simulink model "QPTest5"  (R2021a)
settings: Solver=ode45  StartTime=0.0  StopTime=20  FixedStep=Control_timestep  RelTol=1e-3  AbsTol=1e-6
undefined symbols (not defined in the file): Matlab_version, NXMotion, NXMotion_controltimestep, NXMotion_model, NXMotion_model_n, NXMotion_n, NXMotion_solution, NXMotion_solution_n, Plant_inputs_num, Plant_outputs_num
libraries: simulink x1
(part 1 of 3)
settings Model: ExtModeTrigMode=oneshot  ExtModeArmWhenConnect=off  Creator=djyun  LastModifiedBy=Bec
settings SolverCC: AutoScaleAbsTol=off  AlgebraicLoopSolver=TrustRegion
settings DataIOCC: SaveFormat=Array  SignalLoggingSaveFormat=ModelDataLogs  ReturnWorkspaceOutputs=off
settings OptimizationCC: BooleanDataType=off  InitFltsAndDblsToZero=on  LifeSpan=inf
settings DebuggingCC: SaveWithParameterizedLinksMsg=none  UnderspecifiedInitializationDetection=Classic  MergeDetectMultiDrivingBlocksExec=none  SignalResolutionControl=TryResolveAllWithWarning  MultiTaskDSMMsg=warning  MultiTaskCondExecSysMsg=none  FcnCallInpInsideContextMsg=warning  SFUnexpectedBacktrackingDiag=warning  SFNoUnconditionalDefaultTransitionDiag=warning  SFExecutionAtInitializationDiag=none  SFMachineParentedDataDiag=warning  ArithmeticOperatorsInVariantConditions=warning
settings HardwareCC: ProdBitPerPointer=32  ProdBitPerSizeT=32  ProdBitPerPtrDiffT=32  ProdLargestAtomicFloat=None  ProdIntDivRoundTo=Undefined  ProdEndianess=Unspecified  ProdWordSize=32  ProdHWDeviceType=32-bit Generic  TargetUnknown=on
settings ModelReferenceCC: PropagateSignalLabelsOutOfModel=off
settings RTWCC: TemplateMakefile=grt_unix.tmf
settings CodeAppCC: StateflowObjectComments=on
settings GRTTargetCC: TargetFcnLib=ansi_tfl_tmw.mat  TargetLangStandard=C89/C90 (ANSI)  ModelReferenceCompliant=off  CombineOutputUpdateFcns=off  MatFileLogging=off  GRTInterface=on
settings ConfigComp: CovMetricSettings=dw  CovSaveCumulativeToWorkspaceVar=on  CovSaveSingleToWorkspaceVar=on

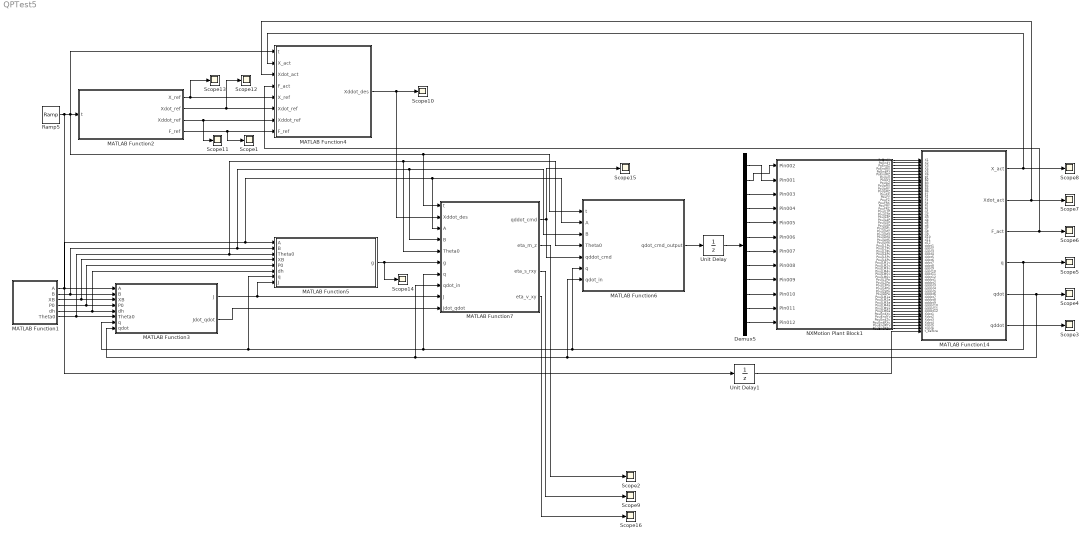
== system QPTest5 ==
  Demux5 : Demux  Outputs=12
  MATLAB Function1 : MATLAB Function  TreatAsAtomicUnit=on
  MATLAB Function14 : MATLAB Function  TreatAsAtomicUnit=on
  MATLAB Function2 : MATLAB Function  TreatAsAtomicUnit=on
  MATLAB Function3 : MATLAB Function  TreatAsAtomicUnit=on
  MATLAB Function4 : MATLAB Function  TreatAsAtomicUnit=on
  MATLAB Function5 : MATLAB Function  TreatAsAtomicUnit=on
  MATLAB Function6 : MATLAB Function  TreatAsAtomicUnit=on
  MATLAB Function7 : MATLAB Function  TreatAsAtomicUnit=on
  NXMotion Plant Block1 : Subsystem
      mask Display: image(imread('NXMOTION_Logo_Client.TIF'))
  Ramp5 : simulink/Sources/Ramp  slope=1  start=0  InitialOutput=0
  Scope{1..16} (16 alike) : Scope
  Unit Delay : UnitDelay  InitialCondition=zeros(12,1)  SampleTime=1e-3  HasFrameUpgradeWarning=on
  Unit Delay1 : UnitDelay  InitialCondition=zeros(1,1)  SampleTime=1e-3  HasFrameUpgradeWarning=on
  wires:
  MATLAB Function2/1(X_ref) -> MATLAB Function4/5(X_ref), Scope13/1
  MATLAB Function2/2(Xdot_ref) -> MATLAB Function4/6(Xdot_ref), Scope12/1
  MATLAB Function2/3(Xddot_ref) -> MATLAB Function4/7(Xddot_ref), Scope11/1
  MATLAB Function7/1(qddot_cmd) -> Scope15/1, MATLAB Function6/5(qddot_cmd)
  MATLAB Function2/4(F_ref) -> MATLAB Function4/8(F_ref), Scope1/1
  MATLAB Function3/1(J) -> MATLAB Function5/8(J), MATLAB Function7/9(J)
  MATLAB Function3/2(Jdot_qdot) -> MATLAB Function7/10(Jdot_qdot)
  MATLAB Function4/1(Xddot_des) -> Scope10/1, MATLAB Function7/2(Xddot_des)
  MATLAB Function5/1(g) -> Scope14/1, MATLAB Function7/6(g)
  MATLAB Function1/1(A) -> MATLAB Function3/1(A), MATLAB Function6/2(A), MATLAB Function7/3(A), MATLAB Function5/1(A)
  MATLAB Function1/2(B) -> MATLAB Function6/3(B), MATLAB Function7/4(B), MATLAB Function5/2(B), MATLAB Function3/2(B)
  MATLAB Function1/3(XB) -> MATLAB Function5/4(XB), MATLAB Function3/3(XB)
  MATLAB Function1/4(P0) -> MATLAB Function5/5(P0), MATLAB Function3/4(P0)
  MATLAB Function1/5(dh) -> MATLAB Function5/6(dh), MATLAB Function3/5(dh)
  MATLAB Function1/6(Theta0) -> MATLAB Function6/4(Theta0), MATLAB Function7/5(Theta0), MATLAB Function5/3(Theta0), MATLAB Function3/6(Theta0)
  MATLAB Function6/1(qdot_cmd_output) -> Unit Delay/1
  Unit Delay/1 -> Demux5/1
  MATLAB Function14/1(X_act) -> Scope8/1, MATLAB Function4/2(X_act)
  MATLAB Function14/2(Xdot_act) -> Scope7/1, MATLAB Function4/3(Xdot_act)
  MATLAB Function14/3(F_act) -> Scope6/1, MATLAB Function4/4(F_act)
  MATLAB Function14/4(q) -> MATLAB Function3/7(q), MATLAB Function5/7(q), MATLAB Function7/7(q), MATLAB Function6/6(q), Scope5/1
  MATLAB Function14/5(qdot) -> MATLAB Function7/8(qdot_in), MATLAB Function3/8(qdot), MATLAB Function6/7(qdot_in), Scope4/1
  MATLAB Function14/6(qddot) -> Scope3/1
  Demux5/3 -> NXMotion Plant Block1/3(Pin003)
  Demux5/4 -> NXMotion Plant Block1/4(Pin004)
  Demux5/5 -> NXMotion Plant Block1/5(Pin005)
  Demux5/6 -> NXMotion Plant Block1/6(Pin006)
  Demux5/7 -> NXMotion Plant Block1/7(Pin007)
  Demux5/8 -> NXMotion Plant Block1/8(Pin008)
  Demux5/9 -> NXMotion Plant Block1/9(Pin009)
  Demux5/10 -> NXMotion Plant Block1/10(Pin010)
  Demux5/11 -> NXMotion Plant Block1/11(Pin011)
  Demux5/12 -> NXMotion Plant Block1/12(Pin012)
  Demux5/2 -> NXMotion Plant Block1/1(Pin002)
  Demux5/1 -> NXMotion Plant Block1/2(Pin001)
  Ramp5/1 -> Unit Delay1/1, MATLAB Function6/1(t), MATLAB Function7/1(t), MATLAB Function2/1(t), MATLAB Function4/1(t)
  NXMotion Plant Block1/1("PoEndX   ") -> MATLAB Function14/1(X1)
  NXMotion Plant Block1/2("PoEndY   ") -> MATLAB Function14/2(X2)
  NXMotion Plant Block1/3("PoEndZ   ") -> MATLAB Function14/3(X3)
  NXMotion Plant Block1/4("PoEndRX  ") -> MATLAB Function14/4(X4)
  NXMotion Plant Block1/5("PoEndRY  ") -> MATLAB Function14/5(X5)
  NXMotion Plant Block1/6("PoEndRZ  ") -> MATLAB Function14/6(X6)
  NXMotion Plant Block1/7("PoUpX    ") -> MATLAB Function14/7(B1)
  NXMotion Plant Block1/8("PoUpY    ") -> MATLAB Function14/8(B2)
  NXMotion Plant Block1/9("PoUpZ    ") -> MATLAB Function14/9(B3)
  NXMotion Plant Block1/10("PoUpRX   ") -> MATLAB Function14/10(B4)
  NXMotion Plant Block1/11("PoUpRY   ") -> MATLAB Function14/11(B5)
  NXMotion Plant Block1/12("PoUpRZ   ") -> MATLAB Function14/12(B6)
  NXMotion Plant Block1/13("PouFX    ") -> MATLAB Function14/13(F1)
  NXMotion Plant Block1/14("PouFY    ") -> MATLAB Function14/14(F2)
  NXMotion Plant Block1/15("PouFZ    ") -> MATLAB Function14/15(F3)
  NXMotion Plant Block1/16("PouFRX   ") -> MATLAB Function14/16(F4)
  NXMotion Plant Block1/17("PouFRY   ") -> MATLAB Function14/17(F5)
  NXMotion Plant Block1/18("PouFRZ   ") -> MATLAB Function14/18(F6)
  NXMotion Plant Block1/19("PouJL1P  ") -> MATLAB Function14/19(q1)
  NXMotion Plant Block1/20("PouJL2P  ") -> MATLAB Function14/20(q2)
  NXMotion Plant Block1/21("PouJL3P  ") -> MATLAB Function14/21(q3)
  NXMotion Plant Block1/22("PouJL4P  ") -> MATLAB Function14/22(q4)
  NXMotion Plant Block1/23("PouJL5P  ") -> MATLAB Function14/23(q5)
  NXMotion Plant Block1/24("PouJL6P  ") -> MATLAB Function14/24(q6)
  NXMotion Plant Block1/25("PouJLM1  ") -> MATLAB Function14/25(q7)
  NXMotion Plant Block1/26("PouJLM2  ") -> MATLAB Function14/26(q8)
  NXMotion Plant Block1/27("PouJLM3  ") -> MATLAB Function14/27(q9)
  NXMotion Plant Block1/28("PouJLM4  ") -> MATLAB Function14/28(q10)
  NXMotion Plant Block1/29("PouJLM5  ") -> MATLAB Function14/29(q11)
  NXMotion Plant Block1/30("PouJLM6  ") -> MATLAB Function14/30(q12)
  NXMotion Plant Block1/31("PouJL1Pv ") -> MATLAB Function14/31(qdot1)
  NXMotion Plant Block1/32("PouJL2Pv ") -> MATLAB Function14/32(qdot2)
  NXMotion Plant Block1/33("PouJL3Pv ") -> MATLAB Function14/33(qdot3)
  NXMotion Plant Block1/34("PouJL4Pv ") -> MATLAB Function14/34(qdot4)
  NXMotion Plant Block1/35("PouJL5Pv ") -> MATLAB Function14/35(qdot5)
  NXMotion Plant Block1/36("PouJL6Pv ") -> MATLAB Function14/36(qdot6)
  NXMotion Plant Block1/37("PouJLM1v ") -> MATLAB Function14/37(qdot7)
  NXMotion Plant Block1/38("PouJLM2v ") -> MATLAB Function14/38(qdot8)
  NXMotion Plant Block1/39("PouJLM3v ") -> MATLAB Function14/39(qdot9)
  NXMotion Plant Block1/40("PouJLM4v ") -> MATLAB Function14/40(qdot10)
  NXMotion Plant Block1/41("PouJLM5v ") -> MATLAB Function14/41(qdot11)
  NXMotion Plant Block1/42("PouJLM6v ") -> MATLAB Function14/42(qdot12)
  NXMotion Plant Block1/43("PouJL1Pa ") -> MATLAB Function14/43(qddot1)
  NXMotion Plant Block1/44("PouJL2Pa ") -> MATLAB Function14/44(qddot2)
  NXMotion Plant Block1/45("PouJL3Pa ") -> MATLAB Function14/45(qddot3)
  NXMotion Plant Block1/46("PouJL4Pa ") -> MATLAB Function14/46(qddot4)
  NXMotion Plant Block1/47("PouJL5Pa ") -> MATLAB Function14/47(qddot5)
  NXMotion Plant Block1/48("PouJL6Pa ") -> MATLAB Function14/48(qddot6)
  NXMotion Plant Block1/49("PouJLM1a ") -> MATLAB Function14/49(qddot7)
  NXMotion Plant Block1/50("PouJLM2a ") -> MATLAB Function14/50(qddot8)
  NXMotion Plant Block1/51("PouJLM3a ") -> MATLAB Function14/51(qddot9)
  NXMotion Plant Block1/52("PouJLM4a ") -> MATLAB Function14/52(qddot10)
  NXMotion Plant Block1/53("PouJLM5a ") -> MATLAB Function14/53(qddot11)
  NXMotion Plant Block1/54("PouJLM6a ") -> MATLAB Function14/54(qddot12)
  NXMotion Plant Block1/55("PouEndXv ") -> MATLAB Function14/55(Xdot1)
  NXMotion Plant Block1/56("PouEndYv ") -> MATLAB Function14/56(Xdot2)
  NXMotion Plant Block1/57("PouEndZv ") -> MATLAB Function14/57(Xdot3)
  NXMotion Plant Block1/58(PouEndRXv) -> MATLAB Function14/58(Xdot4)
  NXMotion Plant Block1/59(PouEndRYv) -> MATLAB Function14/59(Xdot5)
  NXMotion Plant Block1/60(PouEndRZv) -> MATLAB Function14/60(Xdot6)
  Unit Delay1/1 -> MATLAB Function14/61(t_before)
  MATLAB Function7/3(eta_s_rxy) -> Scope9/1
  MATLAB Function7/4(eta_v_xy) -> Scope16/1
  MATLAB Function7/2(eta_m_z) -> Scope2/1

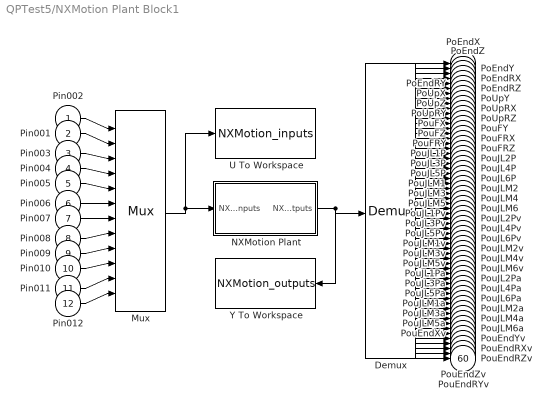
== system QPTest5/NXMotion Plant Block1 ==
  Pin002 : Inport
  Pin001 : Inport  Port=2
  Pin003 : Inport  Port=3
  Pin004 : Inport  Port=4
  Pin005 : Inport  Port=5
  Pin006 : Inport  Port=6
  Pin007 : Inport  Port=7
  Pin008 : Inport  Port=8
  Pin009 : Inport  Port=9
  Pin010 : Inport  Port=10
  Pin011 : Inport  Port=11
  Pin012 : Inport  Port=12
  Demux : Demux  Outputs=60
      settings: DisplayOption=none
  Mux : Mux  Inputs=12
  NXMotion Plant : Subsystem  mask(NXMotion/Plant){NXMotion_model_name=NXMotion_model, NXMotion_=NXMotion, Matlab_version_=Matlab_version, NXMotion_controltimestep_=NXMotion_controltimestep, NXMotion_step_=100, Waitingtime=1000, NXMotion_static_=off}
      mask prompts: NXMotion_ "NXMotion_install_directory"; Matlab_version_ "Matlab version"; NXMotion_controltimestep_ "Sampling period"; NXMotion_step_ "NXMotion_step"; Waitingtime "Waiting time"; NXMotion_static_ "Static analysis"
      mask help:
      | Simulate any NXMotion Model in NXMotion/Solver
      | Plant inputs and Plant outputs are transfered every sampling time
      | Here, sampling time is determined by sampling period (Control time step)
      mask Display: disp( 'Dynamic Model' )
  U To Workspace : ToWorkspace  VariableName=NXMotion_inputs
  Y To Workspace : ToWorkspace  VariableName=NXMotion_outputs
  "PoEndX   " : Outport
  "PoEndY   " : Outport  Port=2
  "PoEndZ   " : Outport  Port=3
  "PoEndRX  " : Outport  Port=4
  "PoEndRY  " : Outport  Port=5
  "PoEndRZ  " : Outport  Port=6
  "PoUpX    " : Outport  Port=7
  "PoUpY    " : Outport  Port=8
  "PoUpZ    " : Outport  Port=9
  "PoUpRX   " : Outport  Port=10
  "PoUpRY   " : Outport  Port=11
  "PoUpRZ   " : Outport  Port=12
  "PouFX    " : Outport  Port=13
  "PouFY    " : Outport  Port=14
  "PouFZ    " : Outport  Port=15
  "PouFRX   " : Outport  Port=16
  "PouFRY   " : Outport  Port=17
  "PouFRZ   " : Outport  Port=18
  "PouJL1P  " : Outport  Port=19
  "PouJL2P  " : Outport  Port=20
  "PouJL3P  " : Outport  Port=21
  "PouJL4P  " : Outport  Port=22
  "PouJL5P  " : Outport  Port=23
  "PouJL6P  " : Outport  Port=24
  "PouJLM1  " : Outport  Port=25
  "PouJLM2  " : Outport  Port=26
  "PouJLM3  " : Outport  Port=27
  "PouJLM4  " : Outport  Port=28
  "PouJLM5  " : Outport  Port=29
  "PouJLM6  " : Outport  Port=30
  "PouJL1Pv " : Outport  Port=31
  "PouJL2Pv " : Outport  Port=32
  "PouJL3Pv " : Outport  Port=33
  "PouJL4Pv " : Outport  Port=34
  "PouJL5Pv " : Outport  Port=35
  "PouJL6Pv " : Outport  Port=36
  "PouJLM1v " : Outport  Port=37
  "PouJLM2v " : Outport  Port=38
  "PouJLM3v " : Outport  Port=39
  "PouJLM4v " : Outport  Port=40
  "PouJLM5v " : Outport  Port=41
  "PouJLM6v " : Outport  Port=42
  "PouJL1Pa " : Outport  Port=43
  "PouJL2Pa " : Outport  Port=44
  "PouJL3Pa " : Outport  Port=45
  "PouJL4Pa " : Outport  Port=46
  "PouJL5Pa " : Outport  Port=47
  "PouJL6Pa " : Outport  Port=48
  "PouJLM1a " : Outport  Port=49
  "PouJLM2a " : Outport  Port=50
  "PouJLM3a " : Outport  Port=51
  "PouJLM4a " : Outport  Port=52
  "PouJLM5a " : Outport  Port=53
  "PouJLM6a " : Outport  Port=54
  "PouEndXv " : Outport  Port=55
  "PouEndYv " : Outport  Port=56
  "PouEndZv " : Outport  Port=57
  PouEndRXv : Outport  Port=58
  PouEndRYv : Outport  Port=59
  PouEndRZv : Outport  Port=60
  wires:
  Pin012/1 -> Mux/12
  Pin011/1 -> Mux/11
  Pin010/1 -> Mux/10
  Pin009/1 -> Mux/9
  Pin008/1 -> Mux/8
  Pin007/1 -> Mux/7
  Pin006/1 -> Mux/6
  Pin005/1 -> Mux/5
  Pin004/1 -> Mux/4
  Pin003/1 -> Mux/3
  Pin001/1 -> Mux/2
  Pin002/1 -> Mux/1
  Demux/60 -> PouEndRZv/1
  Demux/59 -> PouEndRYv/1
  Demux/58 -> PouEndRXv/1
  Demux/57 -> "PouEndZv "/1
  Demux/56 -> "PouEndYv "/1
  Demux/55 -> "PouEndXv "/1
  Demux/54 -> "PouJLM6a "/1
  Demux/53 -> "PouJLM5a "/1
  Demux/52 -> "PouJLM4a "/1
  Demux/51 -> "PouJLM3a "/1
  Demux/50 -> "PouJLM2a "/1
  Demux/49 -> "PouJLM1a "/1
  Demux/48 -> "PouJL6Pa "/1
  Demux/47 -> "PouJL5Pa "/1
  Demux/46 -> "PouJL4Pa "/1
  Demux/45 -> "PouJL3Pa "/1
  Demux/44 -> "PouJL2Pa "/1
  Demux/43 -> "PouJL1Pa "/1
  Demux/42 -> "PouJLM6v "/1
  Demux/41 -> "PouJLM5v "/1
  Demux/40 -> "PouJLM4v "/1
  Demux/39 -> "PouJLM3v "/1
  Demux/38 -> "PouJLM2v "/1
  Demux/37 -> "PouJLM1v "/1
  Demux/36 -> "PouJL6Pv "/1
  Demux/35 -> "PouJL5Pv "/1
  Demux/34 -> "PouJL4Pv "/1
  Demux/33 -> "PouJL3Pv "/1
  Demux/32 -> "PouJL2Pv "/1
  Demux/31 -> "PouJL1Pv "/1
  Demux/30 -> "PouJLM6  "/1
  Demux/29 -> "PouJLM5  "/1
  Demux/28 -> "PouJLM4  "/1
  Demux/27 -> "PouJLM3  "/1
  Demux/26 -> "PouJLM2  "/1
  Demux/25 -> "PouJLM1  "/1
  Demux/24 -> "PouJL6P  "/1
  Demux/23 -> "PouJL5P  "/1
  Demux/22 -> "PouJL4P  "/1
  Demux/21 -> "PouJL3P  "/1
  Demux/20 -> "PouJL2P  "/1
  Demux/19 -> "PouJL1P  "/1
  Demux/18 -> "PouFRZ   "/1
  Demux/17 -> "PouFRY   "/1
  Demux/16 -> "PouFRX   "/1
  Demux/15 -> "PouFZ    "/1
  Demux/14 -> "PouFY    "/1
  Demux/13 -> "PouFX    "/1
  Demux/12 -> "PoUpRZ   "/1
  Demux/11 -> "PoUpRY   "/1
  Demux/10 -> "PoUpRX   "/1
  Demux/9 -> "PoUpZ    "/1
  Demux/8 -> "PoUpY    "/1
  Demux/7 -> "PoUpX    "/1
  Demux/6 -> "PoEndRZ  "/1
  Demux/5 -> "PoEndRY  "/1
  Demux/4 -> "PoEndRX  "/1
  Demux/3 -> "PoEndZ   "/1
  Demux/2 -> "PoEndY   "/1
  Demux/1 -> "PoEndX   "/1
  Mux/1 -> U To Workspace/1, NXMotion Plant/1(NXMotion_inputs)
  NXMotion Plant/1(NXMotion_outputs) -> Y To Workspace/1, Demux/1

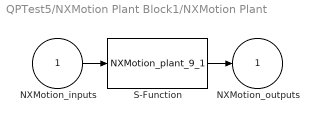
== system QPTest5/NXMotion Plant Block1/NXMotion Plant ==
  NXMotion_inputs : Inport
  S-Function : S-Function  FunctionName=NXMotion_plant_9_1  Parameters=NXMotion_controltimestep_,NXMotion_model_name,NXMotion_,NXMotion_solution,NXMotion_static_,NXMotion_step_,Matlab_version_,NXMotion_model_n,NXMotion_n,NXMotion_solution_n,Plant_inputs_num,Plant_outputs_num,Waitingtime  SFunctionDeploymentMode=off  EnableBusSupport=off
  NXMotion_outputs : Outport  InitialOutput=0
  wires:
  NXMotion_inputs/1 -> S-Function/1
  S-Function/1 -> NXMotion_outputs/1

== matlab function QPTest5/MATLAB Function2 ==
  data: X_ref output; Xdot_ref output; Xddot_ref output; F_ref output; t input
function [X_ref, Xdot_ref, Xddot_ref, F_ref] = Task_Reference(t)

% 输入：
%   t          Ramp 输出的时间信号，单位 s
%
% 输出：
%   X_ref      6x1  末端参考位姿 [x; y; z; alpha; beta; gamma]
%               位置单位：mm
%               姿态单位：deg
%
%   Xdot_ref   6x1  末端参考速度
%               前 3 维单位：mm/s
%               后 3 维单位：deg/s
%
%   Xddot_ref  6x1  末端参考加速度
%               前 3 维单位：mm/s^2
%               后 3 维单位：deg/s^2
%
%   F_ref      6x1  末端参考力/力矩 [Fx; Fy; Fz; Mx; My; Mz]
%               力单位：N
%               力矩单位：N*mm 或与 NX 输出保持一致
%
% traj_mode:
%   traj_mode = 0 : 沿 x 轴直线轨迹
%   traj_mode = 2 : 正方形轨迹
%   traj_mode = 3 : 圆形轨迹
%   traj_mode = 4 : 沿 y 方向前进的三角函数波浪轨迹

    %% -----------------------------
    % 1. 固定输出尺寸
    % ------------------------------
    X_ref     = zeros(6,1);
    Xdot_ref  = zeros(6,1);
    Xddot_ref = zeros(6,1);
    F_ref     = zeros(6,1);

    %% -----------------------------
    % 2. 轨迹模式选择
    %
    %   0 : 直线
    %   2 : 正方形
    %   3 : 圆形
    %   4 : y 方向波浪轨迹
    % ------------------------------
    traj_mode = 2;    

    T_total = 20.0;                 % s
    path_length = 600.0;            % mm

    F_ref_z = 50;
    
    %% -----------------------------
    % 3. 末端初始参考位姿
    % ------------------------------
    X0 = [
        -1161.7884;     % x0, mm
            0.0000;     % y0, mm
         1560.2205;     % z0, mm
            0.0000;     % alpha0, deg
            0.0000;     % beta0,  deg
            0.0000      % gamma0, deg
    ];

    %% -----------------------------
    % 4. 轨迹启动延迟
    % ------------------------------
    t_start = 0.002;     % s

    % 有效轨迹时间
    t_eff = t - t_start;

    %% -----------------------------
    % 5. 总轨迹时间
    %
    % T_traj = T_total - t_start 表示：
    %   轨迹从 t_start 开始，
    %   并在 t = T_total 时结束。
    % ------------------------------
    T_traj  = T_total - t_start;   % s

    if T_traj <= 1.0e-6
        T_traj = 1.0e-6;
    end

    %% -----------------------------
    % 6. 轨迹尺寸参数
    % ------------------------------
    line_length = -path_length;              % mm，负号表示沿世界 -x 方向

    square_side = path_length / 4.0;         % mm

    circle_radius = path_length / (2.0*pi);  % mm

    % y 方向波浪轨迹参数
    wave_y_length = path_length;             % mm，沿 +y 方向前进距离
    wave_amp_x    = 30.0;                    % mm，x 方向波浪振幅
    wave_cycles   = 2.0;                     % 波浪周期数，建议取整数，保证末端回到中心线

    %% -----------------------------
    % 7. 输出位置、速度、加速度初始化
    % ------------------------------
    pos = X0(1:3);
    vel = zeros(3,1);
    acc = zeros(3,1);

    %% =================================================
    % 8. traj_mode = 0：直线轨迹
    %% =================================================
    if traj_mode == 0

        % 直线方向：世界坐标系 +x。
        % 由于 line_length = -200，因此实际运动方向为 -x。
        line_dir = [
            1.0;
            0.0;
            0.0
        ];

        line_dir = line_dir / max(norm(line_dir), 1.0e-12);

        % 五次多项式进度
        if t_eff <= 0.0
            tau = 0.0;
        elseif t_eff >= T_traj
            tau = 1.0;
        else
            tau = t_eff / T_traj;
        end

        tau2 = tau * tau;
        tau3 = tau2 * tau;
        tau4 = tau3 * tau;
        tau5 = tau4 * tau;

        sigma = 10.0*tau3 - 15.0*tau4 + 6.0*tau5;

        if t_eff <= 0.0 || t_eff >= T_traj
            sigma_dot  = 0.0;
            sigma_ddot = 0.0;
        else
            sigma_dot  = (30.0*tau2 - 60.0*tau3 + 30.0*tau4) / T_traj;
            sigma_ddot = (60.0*tau - 180.0*tau2 + 120.0*tau3) / (T_traj*T_traj);
        end

        s     = line_length * sigma;
        sdot  = line_length * sigma_dot;
        sddot = line_length * sigma_ddot;

        pos = X0(1:3) + line_dir * s;
        vel = line_dir * sdot;
        acc = line_dir * sddot;

    %% =================================================
    % 9. traj_mode = 2：正方形轨迹
    %% =================================================
    elseif traj_mode == 2

        % 正方形从 X0 出发，运动顺序：
        %   第 1 边：沿 -x
        %   第 2 边：沿 +y
        %   第 3 边：沿 +x
        %   第 4 边：沿 -y
        % 最后回到 X0。
        T_side = T_traj / 4.0;

        if T_side <= 1.0e-6
            T_side = 1.0e-6;
        end

        p_start = X0(1:3);
        dir = zeros(3,1);
        tau = 0.0;

        if t_eff <= 0.0

            p_start = X0(1:3);
            dir = zeros(3,1);
            tau = 0.0;

        elseif t_eff >= T_traj

            % 正方形闭合，结束后回到 X0 并保持
            p_start = X0(1:3);
            dir = zeros(3,1);
            tau = 0.0;

        else

            seg_id = floor(t_eff / T_side) + 1;

            if seg_id < 1
                seg_id = 1;
            elseif seg_id > 4
                seg_id = 4;
            end

            t_seg = t_eff - double(seg_id - 1) * T_side;
            tau = t_seg / T_side;

            if tau < 0.0
                tau = 0.0;
            elseif tau > 1.0
                tau = 1.0;
            end

            if seg_id == 1

                % X0 -> X0 + [-L; 0; 0]
                p_start = X0(1:3);
                dir = [
                    -1.0;
                     0.0;
                     0.0
                ];

            elseif seg_id == 2

                % X0 + [-L; 0; 0] -> X0 + [-L; L; 0]
                p_start = X0(1:3) + [
                    -square_side;
                     0.0;
                     0.0
                ];

                dir = [
                     0.0;
                     1.0;
                     0.0
                ];

            elseif seg_id == 3

                % X0 + [-L; L; 0] -> X0 + [0; L; 0]
                p_start = X0(1:3) + [
                    -square_side;
                     square_side;
                     0.0
                ];

                dir = [
                     1.0;
                     0.0;
                     0.0
                ];

            else

                % X0 + [0; L; 0] -> X0
                p_start = X0(1:3) + [
                     0.0;
                     square_side;
                     0.0
                ];

                dir = [
                     0.0;
                    -1.0;
                     0.0
                ];

            end
        end

        % 每条边使用五次多项式。
        % 每个拐角处速度和加速度都为 0，避免速度方向突变。
        tau2 = tau * tau;
        tau3 = tau2 * tau;
        tau4 = tau3 * tau;
        tau5 = tau4 * tau;

        sigma = 10.0*tau3 - 15.0*tau4 + 6.0*tau5;

        if t_eff <= 0.0 || t_eff >= T_traj
            sigma_dot  = 0.0;
            sigma_ddot = 0.0;
        else
            sigma_dot  = (30.0*tau2 - 60.0*tau3 + 30.0*tau4) / T_side;
            sigma_ddot = (60.0*tau - 180.0*tau2 + 120.0*tau3) / (T_side*T_side);
        end

        s     = square_side * sigma;
        sdot  = square_side * sigma_dot;
        sddot = square_side * sigma_ddot;

        pos = p_start + dir * s;
        vel = dir * sdot;
        acc = dir * sddot;

    %% =================================================
    % 10. traj_mode = 3：圆形轨迹
    %% =================================================
    elseif traj_mode == 3

        % 圆形轨迹从 X0 出发，并最终回到 X0。
        %
        % 这里设定圆心在 X0 的 -y 方向：
        %   center = X0 + [0; -R; 0]
        %
        % 初始角度 theta0 = pi/2，
        % 因此初始点为：
        %   center + R*[cos(pi/2); sin(pi/2); 0] = X0
        %
        % theta 增大时，初始切向速度沿 -x 方向，
        % 与直线、正方形轨迹的起始方向一致。

        R_c = circle_radius;

        center = X0(1:3) + [
             0.0;
            -R_c;
             0.0
        ];

        theta0 = pi / 2.0;

        % 五次多项式控制整圈角度进度
        if t_eff <= 0.0
            tau = 0.0;
        elseif t_eff >= T_traj
            tau = 1.0;
        else
            tau = t_eff / T_traj;
        end

        tau2 = tau * tau;
        tau3 = tau2 * tau;
        tau4 = tau3 * tau;
        tau5 = tau4 * tau;

        sigma = 10.0*tau3 - 15.0*tau4 + 6.0*tau5;

        if t_eff <= 0.0 || t_eff >= T_traj
            sigma_dot  = 0.0;
            sigma_ddot = 0.0;
        else
            sigma_dot  = (30.0*tau2 - 60.0*tau3 + 30.0*tau4) / T_traj;
            sigma_ddot = (60.0*tau - 180.0*tau2 + 120.0*tau3) / (T_traj*T_traj);
        end

        theta      = theta0 + 2.0*pi*sigma;
        theta_dot  = 2.0*pi*sigma_dot;
        theta_ddot = 2.0*pi*sigma_ddot;

        cth = cos(theta);
        sth = sin(theta);

        % 位置
        pos = center + R_c * [
            cth;
            sth;
            0.0
        ];

        % 速度
        vel = R_c * theta_dot * [
            -sth;
             cth;
             0.0
        ];

        % 加速度：
        % d/dt {R*theta_dot*[-sin(theta); cos(theta)]}
        acc = R_c * theta_ddot * [
            -sth;
             cth;
             0.0
        ] + R_c * theta_dot * theta_dot * [
            -cth;
            -sth;
             0.0
        ];

        % 轨迹结束后强制回到 X0，避免数值误差导致最后一点有极小偏差
        if t_eff >= T_traj
            pos = X0(1:3);
            vel = zeros(3,1);
            acc = zeros(3,1);
        end

    %% =================================================
    % 11. traj_mode = 4：沿 y 方向的三角函数波浪轨迹
    %% =================================================
    elseif traj_mode == 4

        % 波浪轨迹说明：
        %   末端整体沿世界坐标系 +y 方向前进；
        %   同时 x 方向做正弦摆动，形成 x-y 平面内的波浪形轨迹；
        %   z 保持不变，姿态保持不变。
        %
        % 轨迹形式：
        %   y = wave_y_length * sigma
        %   x = wave_amp_x * sin(2*pi*wave_cycles*sigma)
        %
        % 其中 sigma 使用五次多项式，从 0 平滑变化到 1。
        % 因此轨迹起点和终点速度、加速度均为 0。
        %
        % 若希望沿 -y 方向前进，将 wave_y_length 改为负值即可。
        % 若希望波浪更明显，增大 wave_amp_x。
        % 若希望波浪周期更多，增大 wave_cycles。

        if t_eff <= 0.0
            tau = 0.0;
        elseif t_eff >= T_traj
            tau = 1.0;
        else
            tau = t_eff / T_traj;
        end

        tau2 = tau * tau;
        tau3 = tau2 * tau;
        tau4 = tau3 * tau;
        tau5 = tau4 * tau;

        sigma = 10.0*tau3 - 15.0*tau4 + 6.0*tau5;

        if t_eff <= 0.0 || t_eff >= T_traj
            sigma_dot  = 0.0;
            sigma_ddot = 0.0;
        else
            sigma_dot  = (30.0*tau2 - 60.0*tau3 + 30.0*tau4) / T_traj;
            sigma_ddot = (60.0*tau - 180.0*tau2 + 120.0*tau3) / (T_traj*T_traj);
        end

        phase = 2.0 * pi * wave_cycles * sigma;

        phase_dot  = 2.0 * pi * wave_cycles * sigma_dot;
        phase_ddot = 2.0 * pi * wave_cycles * sigma_ddot;

        % 位置
        x_wave = wave_amp_x * sin(phase);
        y_wave = wave_y_length * sigma;

        pos = X0(1:3) + [
            x_wave;
            y_wave;
            0.0
        ];

        % 速度
        xdot_wave = wave_amp_x * cos(phase) * phase_dot;
        ydot_wave = wave_y_length * sigma_dot;

        vel = [
            xdot_wave;
            ydot_wave;
            0.0
        ];

        % 加速度
        xddot_wave = wave_amp_x * ...
            ( -sin(phase) * phase_dot * phase_dot ...
              + cos(phase) * phase_ddot );

        yddot_wave = wave_y_length * sigma_ddot;

        acc = [
            xddot_wave;
            yddot_wave;
            0.0
        ];

        % 轨迹结束后保持最终点
        if t_eff >= T_traj
            pos = X0(1:3) + [
                0.0;
                wave_y_length;
                0.0
            ];

            vel = zeros(3,1);
            acc = zeros(3,1);
        end

    %% =================================================
    % 12. 其他 traj_mode：默认保持 X0
    %% =================================================
    else

        pos = X0(1:3);
        vel = zeros(3,1);
        acc = zeros(3,1);

    end

    %% -----------------------------
    % 13. 参考位姿、速度、加速度输出
    % ------------------------------
    % 位置参考：x-y 平面内轨迹，z 不变
    X_ref(1:3) = pos;

    % 姿态保持不变
    X_ref(4:6) = X0(4:6);

    % 速度参考
    Xdot_ref(1:3) = vel;
    Xdot_ref(4:6) = zeros(3,1);

    % 加速度参考
    Xddot_ref(1:3) = acc;
    Xddot_ref(4:6) = zeros(3,1);

    %% -----------------------------
    % 14. 参考接触力
    % ------------------------------
    F_ref(:) = 0.0;

    if t_eff > 0.0
        % 若 NX 中向下压平面时 F_act(3) 为正，则用 +10。
        % 若 NX 中向下压平面时 F_act(3) 为负，则改成 -10。
        F_ref(3) = F_ref_z;
    else
        F_ref(3) = 0.0;
    end

end

== matlab function QPTest5/MATLAB Function3 ==
  data: A input; B input; XB input; P0 input; dh input; Theta0 input; J output; Jdot_qdot output; q input; qdot input
function [J, Jdot_qdot] = System_Kinematics (A, B, XB, P0, dh, Theta0, q, qdot)
% Stewart(6UPS) + 7R机械臂串并联系统 Jacobian 和 dot(J)*dot(q)
%
% 单位约定：
%   长度：mm
%   角度：deg
%
% q 顺序：
%   q = [l1; ...; l6; theta1; ...; theta7]
%   q(1:6)  ：Stewart 六个电缸绝对长度，mm
%   q(7:13) ：机械臂七个关节角，deg
%   q(13)   ：机械臂第 7 关节固定
%
% 输出：
%   J         6x13，使 Xdot_F = J*qdot13
%             前3行：mm/s；后3行：deg/s
%   Jdot_qdot 6x1，即 dot(J)*qdot13
%             前3行：mm/s^2；后3行：deg/s^2

    %% 0. 输入整理
    J = zeros(6,13);
    Jdot_qdot = zeros(6,1);

    A      = reshape(A,       6, 3);
    B      = reshape(B,       6, 3);
    XB     = reshape(XB,      3, 1);
    P0     = reshape(P0,      3, 1);
    dh     = reshape(dh,      7, 4);
    Theta0 = reshape(Theta0,  7, 1);
    q      = reshape(q,      13, 1);
    qdot   = reshape(qdot,   13, 1);

    deg2rad = pi / 180.0;
    rad2deg = 180.0 / pi;

    %% 1. 构造 qdot13，并强制第 7 机械臂关节速度为 0
    qdot13 = qdot;
    qdot13(13) = 0.0;

    %% 2. 拆分 q 与 qdot
    l_para = q(1:6);             % mm
    q_arm_deg = q(7:13);         % deg

    ldot = qdot13(1:6);          % mm/s
    qdot_arm_deg = qdot13(7:13); % deg/s

    theta7_fixed = Theta0(7);

    q_arm_deg(7) = theta7_fixed;
    qdot_arm_deg(7) = 0.0;

    q_arm_rad = q_arm_deg * deg2rad;
    qdot_arm_rad = qdot_arm_deg * deg2rad;

    %% 3. 几何参数与坐标转换
    A_G0 = A.';             % 3x6
    B_G  = B.';             % 3x6

    XB_G0 = XB(:);          % 3x1
    P0_G  = P0(:);          % 3x1

    A_P = zeros(3,6);
    for i = 1:6
        A_P(:,i) = A_G0(:,i) - P0_G;
    end

    % 机械臂基座 B 相对上平台中心 P 的安装偏置，表达在 {P}
    PpB = XB_G0 - P0_G;     % mm

    PRB = [
        -1.0,  0.0,  0.0;
         0.0, -1.0,  0.0;
         0.0,  0.0,  1.0
    ];

    % dh 中角度列 deg -> rad，长度列保持 mm
    dh_rad = dh;
    dh_rad(:,3) = dh(:,3) * deg2rad;
    dh_rad(:,4) = dh(:,4) * deg2rad;

    %% 4. Stewart 正运动学：由六个电缸长度求当前上平台位姿
    pose_guess_p = P0_G;
    pose_guess_R = eye(3);

    maxIter = 60;
    tol = 1.0e-7;

    [p_GP, R_GP] = stewart_fk_LM( ...
        A_P, B_G, l_para, ...
        pose_guess_p, pose_guess_R, ...
        maxIter, tol);

    %% 5. Stewart 速度雅可比
    [Gq, ~, ~, ~] = stewart_Gq(A_P, B_G, p_GP, R_GP);

    lambda_dls = 1.0e-3;
    A_dls  = Gq.' * Gq + lambda_dls^2 * eye(6);
    J_para = A_dls \ Gq.';

    %% 6. 机械臂 Jacobian，表达在机械臂基坐标系 {B}
    % --------------------------------------------------

    X_AEnd0_G = [-1161.7884; 0.0001; 1560.2205];

    q_arm0_deg = Theta0(:);
    q_arm0_deg(7) = Theta0(7);
    q_arm0_rad = q_arm0_deg * deg2rad;

    % 初始 MDH 末端坐标系 {F} 的位姿，p_tool_F = 0 表示先取 MDH 末端原点
    [~, T_BF0, f_F0_B, ~] = franka_jacobian_mdh_tool( ...
        q_arm0_rad, dh_rad, zeros(3,1));

    R_BF0 = T_BF0(1:3,1:3);

    % 初始时：
    %   X_AEnd0_G = XB_G0 + PRB * (f_F0_B + R_BF0*p_AEnd_F)
    %
    % 因此：
    %   p_AEnd_F = R_BF0' * ( PRB'*(X_AEnd0_G-XB_G0) - f_F0_B )
    p_AEnd_F = R_BF0.' * (PRB.' * (X_AEnd0_G - XB_G0) - f_F0_B);

    % 当前真实控制点 AEnd 的机械臂雅可比
    [J_arm_B_full, ~, f_B, Tlist] = franka_jacobian_mdh_tool( ...
        q_arm_rad, dh_rad, p_AEnd_F);
 
    % 第 7 关节固定：保留其位姿影响，但去掉速度列
    J_arm_B = J_arm_B_full;
    J_arm_B(:,7) = 0.0;

    %% 7. 组合系统总 Jacobian，内部先用 [mm/s; rad/s]
    % ^G R_B = ^G R_P * ^P R_B
    R_B = R_GP * PRB;

    % 从 P 到 AEnd 的向量，表达在 {G}
    r_PF = R_GP * PpB + R_B * f_B;

    G_PF = zeros(6,6);
    G_PF(1:3,1:3) = eye(3);
    G_PF(1:3,4:6) = -skew3(r_PF);
    G_PF(4:6,4:6) = eye(3);

    Rbar_B = zeros(6,6);
    Rbar_B(1:3,1:3) = R_B;
    Rbar_B(4:6,4:6) = R_B;

    J_stew_internal = G_PF  * J_para;
    J_arm_internal  = Rbar_B * J_arm_B;
    J_internal = [J_stew_internal, J_arm_internal];

    D_in = diag([ ...
        1; 1; 1; 1; 1; 1; ...
        deg2rad; deg2rad; deg2rad; deg2rad; deg2rad; deg2rad; deg2rad]);

    D_out = diag([1; 1; 1; rad2deg; rad2deg; rad2deg]);

    J = D_out * J_internal * D_in;
    J(:,13) = 0.0;

    %% 8. 计算 dot(J)*qdot
    % 8.1 Stewart 平台速度
    Xdot_P = J_para * ldot;
    v_P = Xdot_P(1:3);
    w_P = Xdot_P(4:6);

    % 8.2 Stewart 平台 bias 加速度
    dGq_dt  = stewart_dGq_twist(A_P, B_G, p_GP, R_GP, v_P, w_P);
    dJ_para = dls_inverse_dJ(Gq, dGq_dt, lambda_dls, A_dls, J_para);

    Xddot_P = dJ_para * ldot;
    dotv_P = Xddot_P(1:3);
    dotw_P = Xddot_P(4:6);

    % 8.3 机械臂相对 twist 和相对 bias 加速度，表达在 {B}
    Xdot_rel_B = J_arm_B * qdot_arm_rad;
    v_rel_B = Xdot_rel_B(1:3);
    w_rel_B = Xdot_rel_B(4:6);

    Xddot_rel_B = armJdotQdot_geometric_fromTlist_tool( ...
        J_arm_B, Tlist, qdot_arm_rad, f_B);

    dotv_rel_B = Xddot_rel_B(1:3);
    dotw_rel_B = Xddot_rel_B(4:6);

    % 8.4 转到世界坐标系 {G}
    v_rel_G    = R_B * v_rel_B;
    w_rel_G    = R_B * w_rel_B;
    dotv_rel_G = R_B * dotv_rel_B;
    dotw_rel_G = R_B * dotw_rel_B;

    % 8.5 末端 bias 加速度
    dotw_F_internal = dotw_P ...
                    + cross(w_P, w_rel_G) ...
                    + dotw_rel_G;

    dotv_F_internal = dotv_P ...
                    + cross(dotw_P, r_PF) ...
                    + cross(w_P, cross(w_P, r_PF)) ...
                    + 2.0 * cross(w_P, v_rel_G) ...
                    + dotv_rel_G;

    Jdot_qdot_internal = [dotv_F_internal; dotw_F_internal];
    Jdot_qdot = D_out * Jdot_qdot_internal;

    J(:,13) = 0.0;
   
end



%% ========================================================================
%                          Stewart FK: Levenberg-Marquardt
% ========================================================================
function [p, R] = stewart_fk_LM(A_P, B_G, l, p0, R0, maxIter, tol)
% Stewart forward kinematics by LM.
% A_P, B_G, l, p 均为 mm；旋转增量为 rad。

    p = p0(:);
    R = R0;

    lambda = 1.0e-4;
    resPrev = inf;

    for it = 1:maxIter 
        [g, Gq] = stewart_residual_and_Gq(A_P, B_G, p, R, l);
        res = norm(g);

        if res < tol
            break;
        end

        H = Gq.' * Gq + lambda * eye(6);
        delta = -(H \ (Gq.' * g));

        accepted = false;
        for trial = 1:10 
            p_new = p + delta(1:3);
            % 左扰动：delta_phi 为空间角速度/旋转增量，对应 Gq 中 -[R*A]x 项。
            R_new = so3_exp(delta(4:6)) * R;

            g_new = stewart_residual_only(A_P, B_G, p_new, R_new, l);
            res_new = norm(g_new);

            if res_new < res
                p = p_new;
                R = R_new;
                lambda = max(lambda / 5.0, 1.0e-12);
                accepted = true;
                break;
            else
                lambda = lambda * 5.0;
                H = Gq.' * Gq + lambda * eye(6);
                delta = -(H \ (Gq.' * g));
            end
        end

        if ~accepted
            break;
        end

        if abs(resPrev - res) / max(1.0, res) < 1.0e-12
            break;
        end
        resPrev = res;
    end
end

function g = stewart_residual_only(A_P, B_G, p, R, l)
    p = p(:);
    g = zeros(6,1);
    for i = 1:6
        s_i = R * A_P(:,i) + p - B_G(:,i);
        g(i) = norm(s_i) - l(i);
    end
end

function [g, Gq] = stewart_residual_and_Gq(A_P, B_G, p, R, l)
    p = p(:);
    g = zeros(6,1);
    Gq = zeros(6,6);

    rA_G = R * A_P;
    for i = 1:6
        s_i = rA_G(:,i) + p - B_G(:,i);
        L_i = norm(s_i);
        L_i_safe = max(L_i, 1.0e-12);
        u_i = s_i / L_i_safe;

        g(i) = L_i - l(i);
        Gq(i,1:3) = u_i.';
        Gq(i,4:6) = u_i.' * (-skew3(rA_G(:,i)));
    end
end

%% ========================================================================
%                          Stewart velocity Jacobian
% ========================================================================
function [Gq, u_all, rA_G_all, legVec_all] = stewart_Gq(A_P, B_G, p, R)
    p = p(:);

    Gq = zeros(6,6);
    u_all = zeros(3,6);
    rA_G_all = R * A_P;
    legVec_all = zeros(3,6);

    for i = 1:6
        s_i = rA_G_all(:,i) + p - B_G(:,i);
        L_i = norm(s_i);
        L_i_safe = max(L_i, 1.0e-12);
        u_i = s_i / L_i_safe;

        legVec_all(:,i) = s_i;
        u_all(:,i) = u_i;

        Gq(i,1:3) = u_i.';
        Gq(i,4:6) = u_i.' * (-skew3(rA_G_all(:,i)));
    end
end

%% ========================================================================
%                          Franka / 机械臂 MDH Jacobian
% ========================================================================
function [J, T_BF, f_B, Tlist] = franka_jacobian_mdh_tool(q_rad, dh_rad, p_tool_F)

    q_rad = q_rad(:);
    p_tool_F = reshape(p_tool_F, 3, 1);

    theta = q_rad + dh_rad(:,4);

    T = eye(4);
    Tlist = zeros(4,4,7);

    for i = 1:7
        a     = dh_rad(i,1);
        d     = dh_rad(i,2);
        alpha = dh_rad(i,3);
        th    = theta(i);

        Ti = mdh_T(a, d, alpha, th);
        T = T * Ti;
        Tlist(:,:,i) = T;
    end

    T_BF = T;

    R_BF = T_BF(1:3,1:3);
    p_F_B = T_BF(1:3,4);

    % AEnd 点在机械臂基坐标系 {B} 下的位置
    f_B = p_F_B + R_BF * p_tool_F;

    J = zeros(6,7);
    p_e = f_B;

    for i = 1:7
        Ti = Tlist(:,:,i);
        zi = Ti(1:3,3);
        pi = Ti(1:3,4);

        J(1:3,i) = cross(zi, p_e - pi);
        J(4:6,i) = zi;
    end
end

function T = mdh_T(a, d, alpha, theta)
% MDH: Tx(a) * Rx(alpha) * Tz(d) * Rz(theta)
% a,d: mm; alpha,theta: rad
    ca = cos(alpha);
    sa = sin(alpha);
    ct = cos(theta);
    st = sin(theta);

    T = [
        ct,    -st,     0,   a;
        st*ca, ct*ca,  -sa, -d*sa;
        st*sa, ct*sa,   ca,  d*ca;
        0,      0,      0,   1
    ];
end

%% ========================================================================
%                          dot(J_arm)*qdot_arm
% ========================================================================
function Jdotq = armJdotQdot_geometric_fromTlist_tool(J_arm_B, Tlist, qdot_rad, p_e)

    qdot_rad = qdot_rad(:);
    p_e = reshape(p_e, 3, 1);

    n = 7;

    z = zeros(3,n);
    p = zeros(3,n);

    for i = 1:n
        Ti = Tlist(:,:,i);
        z(:,i) = Ti(1:3,3);
        p(:,i) = Ti(1:3,4);
    end

    v_e = J_arm_B(1:3,:) * qdot_rad;

    omega_i = zeros(3,n);
    v_i     = zeros(3,n);

    for i = 1:n
        omega_i(:,i) = z(:,1:i) * qdot_rad(1:i);

        vi = zeros(3,1);
        for k = 1:i
            vi = vi + cross(z(:,k), p(:,i) - p(:,k)) * qdot_rad(k);
        end
        v_i(:,i) = vi;
    end

    vdot_bias = zeros(3,1);
    wdot_bias = zeros(3,1);

    for i = 1:n
        zi = z(:,i);
        pi = p(:,i);

        z_dot = cross(omega_i(:,i), zi);
        wdot_bias = wdot_bias + z_dot * qdot_rad(i);

        vdot_bias = vdot_bias + ...
            ( cross(z_dot, p_e - pi) ...
            + cross(zi, v_e - v_i(:,i)) ) * qdot_rad(i);
    end

    Jdotq = [vdot_bias; wdot_bias];
end

%% ========================================================================
%                          Stewart dGq/dt
% ========================================================================
function dGq = stewart_dGq_twist(A_P, B_G, p, R, v, w)

    p = p(:);
    v = v(:);
    w = w(:);

    dGq = zeros(6,6);
    rA = R * A_P;

    for i = 1:6
        rAi = rA(:,i);
        s_i = rAi + p - B_G(:,i);

        L_i = norm(s_i);
        L_i_safe = max(L_i, 1.0e-12);
        u_i = s_i / L_i_safe;

        ds = v + cross(w, rAi);
        dL = u_i.' * ds;
        du = (ds - u_i * dL) / L_i_safe;

        drAi = cross(w, rAi);

        dGq(i,1:3) = du.';
        dGq(i,4:6) = du.' * (-skew3(rAi)) ...
                   + u_i.' * (-skew3(drAi));
    end
end

%% ========================================================================
%                          DLS inverse derivative
% ========================================================================
function dJ = dls_inverse_dJ(G, dG, lambda_dls, A, J)
% J = inv(G^T G + lambda^2 I)*G^T 的时间导数。
% dJ = A^{-1} dG^T - A^{-1}(dG^T G + G^T dG)J

    if nargin < 4
        A = G.' * G + lambda_dls^2 * eye(size(G,2));
    end
    if nargin < 5
        J = A \ G.';
    end

    dA = dG.' * G + G.' * dG;
    dJ = (A \ dG.') - (A \ (dA * J));
end

%% ========================================================================
%                          Basic SO(3) functions
% ========================================================================
function S = skew3(v)
    v = v(:);
    S = [
          0,   -v(3),  v(2);
        v(3),    0,  -v(1);
       -v(2),  v(1),    0
    ];
end

function R = so3_exp(w)
    w = w(:);
    th = norm(w);

    if th < 1.0e-12
        R = eye(3) + skew3(w);
        return;
    end

    k = w / th;
    K = skew3(k);
    R = eye(3) + sin(th) * K + (1.0 - cos(th)) * (K * K);
end

== matlab function QPTest5/MATLAB Function4 ==
  data: Xddot_des output; t input; X_act input; Xdot_act input; F_act input; X_ref input; Xdot_ref input; Xddot_ref input; F_ref input
function Xddot_des = Force_Motion_Controller( ...
    t, X_act, Xdot_act, F_act, ...
    X_ref, Xdot_ref, Xddot_ref, F_ref)


%% -----------------------------
% 0. 固定输出尺寸与输入整理
% ------------------------------
Xddot_des = zeros(6,1);

X_act     = reshape(X_act,     6, 1);
Xdot_act  = reshape(Xdot_act,  6, 1);
F_act     = reshape(F_act,     6, 1);
X_ref     = reshape(X_ref,     6, 1);
Xdot_ref  = reshape(Xdot_ref,  6, 1);
Xddot_ref = reshape(Xddot_ref, 6, 1);
F_ref     = reshape(F_ref,     6, 1);

%% -----------------------------
% 1. 启动保护
% ------------------------------
t_start = 2.0e-3;   % s

if t < t_start
    Xddot_des(:) = 0.0;
    return;
end

%% -----------------------------
% 2. 控制模式
% ------------------------------
enable_force_control = true;

%% -----------------------------
% 3. 误差定义
% ------------------------------
Delta_F    = F_ref    - F_act;
Delta_X    = X_ref    - X_act;
Delta_Xdot = Xdot_ref - Xdot_act;

% 姿态误差归一化到 [-180 deg, 180 deg]
Delta_X(4) = wrapTo180_deg_local(Delta_X(4));
Delta_X(5) = wrapTo180_deg_local(Delta_X(5));
Delta_X(6) = wrapTo180_deg_local(Delta_X(6));

% NaN / Inf 保护
for i = 1:6
    if ~isfinite(Delta_X(i))
        Delta_X(i) = 0.0;
    end

    if ~isfinite(Delta_Xdot(i))
        Delta_Xdot(i) = 0.0;
    end

    if ~isfinite(Xddot_ref(i))
        Xddot_ref(i) = 0.0;
    end

    if ~isfinite(Delta_F(i))
        Delta_F(i) = 0.0;
    end
end

%% -----------------------------
% 4. 运动 PD 控制参数
% ------------------------------
Kp_x = 25;
Kd_x = 10;

Kp_y = 25;
Kd_y = 10;

Kp_z = 25;
Kd_z = 10;

Kp_ori = 10;
Kd_ori = 6;

Xddot_motion = zeros(6,1);

% x 方向
Xddot_motion(1) = Xddot_ref(1) ...
                + Kp_x * Delta_X(1) ...
                + Kd_x * Delta_Xdot(1);

% y 方向
Xddot_motion(2) = Xddot_ref(2) ...
                + Kp_y * Delta_X(2) ...
                + Kd_y * Delta_Xdot(2);

% z 方向
Xddot_motion(3) = Xddot_ref(3) ...
                + Kp_z * Delta_X(3) ...
                + Kd_z * Delta_Xdot(3);

% 姿态 alpha
Xddot_motion(4) = Xddot_ref(4) ...
                + Kp_ori * Delta_X(4) ...
                + Kd_ori * Delta_Xdot(4);

% 姿态 beta
Xddot_motion(5) = Xddot_ref(5) ...
                + Kp_ori * Delta_X(5) ...
                + Kd_ori * Delta_Xdot(5);

% 姿态 gamma
Xddot_motion(6) = Xddot_ref(6) ...
                + Kp_ori * Delta_X(6) ...
                + Kd_ori * Delta_Xdot(6);

%% -----------------------------
% 5. z 方向力阻抗控制
% ------------------------------
MF_z = 50.0;     % kg
DF_z = 120.0;    % N*s/m
KF_z = 20.0;     % N/m

mm_to_m = 1.0e-3;
m_to_mm = 1.0e3;

Delta_z_m     = Delta_X(3)    * mm_to_m;
Delta_zdot_m  = Delta_Xdot(3) * mm_to_m;
Xddot_ref_z_m = Xddot_ref(3)  * mm_to_m;

Xddot_force_z_m = Xddot_ref_z_m ...
    + (Delta_F(3) - DF_z * Delta_zdot_m - KF_z * Delta_z_m) / MF_z;

Xddot_force_z = Xddot_force_z_m * m_to_mm;

if ~isfinite(Xddot_force_z)
    Xddot_force_z = 0.0;
end

%% -----------------------------
% 6. 合成期望末端加速度
% ------------------------------
if enable_force_control
    % 混合力/位控制：
    %   z 力控，x/y/姿态运动控制
    Xddot_des(1) = Xddot_motion(1);
    Xddot_des(2) = Xddot_motion(2);
    Xddot_des(3) = Xddot_force_z;
    Xddot_des(4) = Xddot_motion(4);
    Xddot_des(5) = Xddot_motion(5);
    Xddot_des(6) = Xddot_motion(6);
else
    % 纯轨迹跟踪：
    %   x/y/z/姿态全部运动控制
    Xddot_des = Xddot_motion;
end

%% -----------------------------
% 7. 调试阶段限幅
% ------------------------------
acc_lim_xyz = 1000.0;   % mm/s^2
acc_lim_ori = 100.0;    % deg/s^2

Xddot_des(1) = sat_scalar_local(Xddot_des(1), -acc_lim_xyz, acc_lim_xyz);
Xddot_des(2) = sat_scalar_local(Xddot_des(2), -acc_lim_xyz, acc_lim_xyz);
Xddot_des(3) = sat_scalar_local(Xddot_des(3), -acc_lim_xyz, acc_lim_xyz);

Xddot_des(4) = sat_scalar_local(Xddot_des(4), -acc_lim_ori, acc_lim_ori);
Xddot_des(5) = sat_scalar_local(Xddot_des(5), -acc_lim_ori, acc_lim_ori);
Xddot_des(6) = sat_scalar_local(Xddot_des(6), -acc_lim_ori, acc_lim_ori);

end

function y = wrapTo180_deg_local(x)
deg2rad = pi / 180.0;
rad2deg = 180.0 / pi;

y = atan2(sin(x * deg2rad), cos(x * deg2rad)) * rad2deg;
end

function y = sat_scalar_local(x, lb, ub)
if ~isfinite(x)
    x = 0.0;
end

y = x;

if y < lb
    y = lb;
end

if y > ub
    y = ub;
end
end
